simulink model "sfcndemo_simomex"  (Simulink 7.6)
settings: Solver=ode5  StartTime=0.0  StopTime=20  RelTol=1e-3
Description:
  | Continuous-Time State-Space C-MEX S-function
settings Model: Creator=The MathWorks Inc.  ExtModeTrigMode=oneshot  ExtModeArmWhenConnect=off  ExtModeAutoUpdateStatusClock=off
settings DataIOCC: LimitDataPoints=off
settings OptimizationCC: BlockReduction=off  BooleanDataType=off  InitFltsAndDblsToZero=on
settings DebuggingCC: SaveWithParameterizedLinksMsg=none  SignalResolutionControl=TryResolveAllWithWarning  SolverPrmCheckMsg=none  MultiTaskDSMMsg=warning  MultiTaskCondExecSysMsg=none
settings HardwareCC: TargetUnknown=on
settings RTWCC: IncludeERTFirstTime=on
settings CodeAppCC: CustomSymbolStrFcn=$F$N$M
settings GRTTargetCC: TargetFcnLib=ansi_tfl_tmw.mat

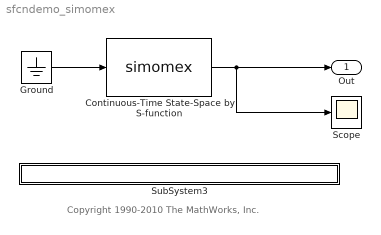
== system sfcndemo_simomex ==
  note: Copyright 1990-2010 The MathWorks, Inc.
  Continuous-Time State-Space by S-function : S-Function  FunctionName=simomex  EnableBusSupport=off
      mask Type: S-function: simomex
      mask Description: This is a S-function block which has single-input and two output state-space system.
      mask Display: disp('dx/dt = A*X + B*U\nY      = C*X + D*U');
  Ground : Ground
  Scope : Scope
  SubSystem3 : Subsystem  mask{filename=simomex.c}
      mask init:
      | x=sfundemo_maskdisp;
      settings: AttributesFormatString=\n  OpenFcn=sfundemo_openfcn
      mask Display: disp(x);
  Out : Outport  InitialOutput=0
  wires:
  Ground/1 -> Continuous-Time State-Space by S-function/1
  Continuous-Time State-Space by S-function/1 -> Out/1, Scope/1

== system sfcndemo_simomex/SubSystem3 ==
